simulink model "slexVariantStopCondProp"  (Simulink 10.0)
settings: Solver=FixedStepAuto  StartTime=0.0  StopTime=10.0  RelTol=1e-3  EnableMultiTasking=on
model workspace (MAT data in the model file):
  V = 1
  W : num (value not decoded)
PreLoadFcn:
  | addpath(fileparts(which(bdroot)));
PostLoadFcn:
  | A = Simulink.Parameter(int32(1));
  | A.StorageClass = 'Define (Custom)';
  | A.CoderInfo.CustomAttributes.HeaderFile='variant_defines.h';
  | 
  | W=copy(A);
settings Model: Creator=The MathWorks, Inc.  LastModifiedBy=bhisma
settings DataIOCC: ReturnWorkspaceOutputs=on  OutputSaveName=out1,out2,out3
settings OptimizationCC: LifeSpan=auto
settings DebuggingCC: UnderspecifiedInitializationDetection=Simplified  MergeDetectMultiDrivingBlocksExec=error  PregeneratedLibrarySubsystemCodeDiagnostic=none  SFUnexpectedBacktrackingDiag=error  SFNoUnconditionalDefaultTransitionDiag=error  SFExecutionAtInitializationDiag=warning
settings HardwareCC: ProdBitPerPointer=64  ProdBitPerSizeT=64  ProdBitPerPtrDiffT=64  ProdLargestAtomicFloat=Float  ProdIntDivRoundTo=Zero  ProdEndianess=LittleEndian  ProdWordSize=64  ProdHWDeviceType=Intel->x86-64 (Windows64)
settings ModelReferenceCC: PropagateSignalLabelsOutOfModel=on
settings RTWCC: SystemTargetFile=ert.tlc  TemplateMakefile=ert_default_tmf
settings GRTTargetCC: CombineOutputUpdateFcns=on  GRTInterface=off
settings ConfigComp: CovMetricSettings=dsw  CovShowResultsExplorer=off  CovExternalEMLEnable=off

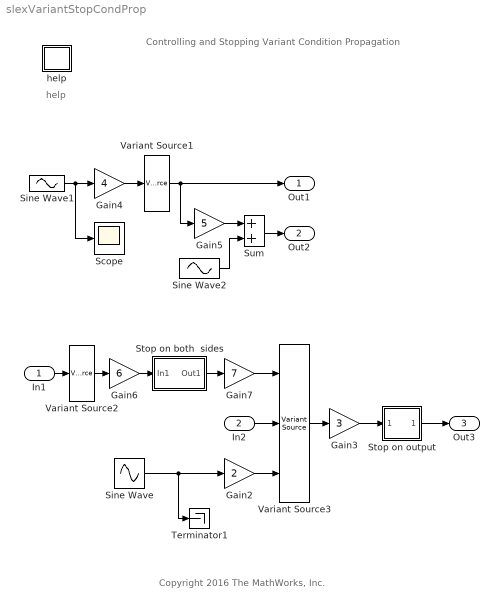
== system slexVariantStopCondProp ==
  note: Controlling and Stopping
      | Variant Condition Propagation
  note: Copyright 2016 The MathWorks, Inc.
  note: help
  In1 : Inport  PortDimensions=1
  In2 : Inport  Port=2  PortDimensions=1
  Gain2 : Gain  Gain=2
  Gain3 : Gain  Gain=3
  Gain4 : Gain  Gain=4
  Gain5 : Gain  Gain=5
  Gain6 : Gain  Gain=6
  Gain7 : Gain  Gain=7
  Scope : Scope
  Sine Wave : Sin  SineType=Sample based  SampleTime=.1
  Sine Wave1 : Sin  SineType=Sample based  SampleTime=.1
  Sine Wave2 : Sin  SineType=Sample based  SampleTime=.1
  Stop on both  sides : Subsystem
  Stop on output : Subsystem
  Sum : Sum
  Terminator1 : Terminator
  Variant Source1 : VariantSource  VariantControls=DataTag1
      settings: GeneratePreprocessorConditionals=on  AllowZeroVariantControls=on
  Variant Source2 : VariantSource  VariantControls=DataTag2
      settings: GeneratePreprocessorConditionals=on  AllowZeroVariantControls=on
  Variant Source3 : VariantSource  VariantControls=DataTag3
      settings: GeneratePreprocessorConditionals=on  AllowZeroVariantControls=on
  help : Subsystem
      mask Display: disp('?')
  Out1 : Outport  VectorParamsAs1DForOutWhenUnconnected=off
  Out2 : Outport  Port=2  VectorParamsAs1DForOutWhenUnconnected=off
  Out3 : Outport  Port=3  VectorParamsAs1DForOutWhenUnconnected=off
  wires:
  Variant Source2/1 -> Gain6/1
  Gain6/1 -> Stop on both  sides/1(In1)
  Stop on both  sides/1(Out1) -> Gain7/1
  Gain7/1 -> Variant Source3/1
  In2/1 -> Variant Source3/2
  Sine Wave/1 -> Terminator1/1, Gain2/1
  Gain2/1 -> Variant Source3/3
  In1/1 -> Variant Source2/1
  Variant Source3/1 -> Gain3/1
  Gain3/1 -> Stop on output/1(In1)
  Stop on output/1(Out1) -> Out3/1
  Sine Wave1/1 -> Gain4/1, Scope/1
  Gain4/1 -> Variant Source1/1
  Sum/1 -> Out2/1
  Sine Wave2/1 -> Sum/2
  Gain5/1 -> Sum/1
  Variant Source1/1 -> Gain5/1, Out1/1

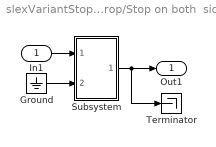
== system slexVariantStopCondProp/Stop on both  sides ==
  In1 : Inport
  Ground : Ground
  Subsystem : Subsystem
  Terminator : Terminator
  Out1 : Outport  VectorParamsAs1DForOutWhenUnconnected=off
  wires:
  In1/1 -> Subsystem/1(In1)
  Ground/1 -> Subsystem/2(In2)
  Subsystem/1(Out1) -> Terminator/1, Out1/1

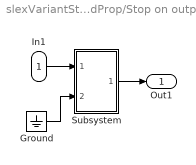
== system slexVariantStopCondProp/Stop on output ==
  In1 : Inport
  Ground : Ground
  Subsystem : Subsystem
  Out1 : Outport  VectorParamsAs1DForOutWhenUnconnected=off
  wires:
  In1/1 -> Subsystem/1(In1)
  Ground/1 -> Subsystem/2(In2)
  Subsystem/1(Out1) -> Out1/1

== system slexVariantStopCondProp/help ==
  note: This illustrates how to control variant condition propagation capabilities of Simulink. Simulink will automatically
      | compute the variant regions based on block connectivity. This is known as variant condition propagation. During
      | variant condition propagation, Simulink automatically assigns conditions to blocks. You can view the conditions
      | assigned to blocks by updating diagram and then looking at the "Display -> Blocks -> Variant Condition Legend".
      |
      | The Variant Source1 has condition, A == 1, which is propagated backwards and forward to the connected blocks. After updating diagram and examining the "Display -> Blocks -> Variant Condition Legend" we see that the Sine Wave1 block is unconditional. This is because the Scope is unconditional and therefore its input, which is the output of the Sine Wave1, must be unconditional. If we were to remove (or comment-out) the Scope, and update diagram we'd see the Sine Wave1 become conditional. Replacing the Scope it with any other block including a Terminator would result in Sine Wave1 being unconditional.
      |
      | We also see that the Sum block is unconditional. This is because the 2nd input to the Sum block is an unconditional signal and therefore the output of the Sum must be unconditional. If we were to place the Gain5, Sum, and Sine Wave2 blocks in a Subsystem (select and ^G) then the Subsystem will be conditional which means the blocks within the Subsystem are also conditional. The subsystem is conditional because it is a system (a well-defined algorithm) with only one input and that input is conditional. If you would like the Subsystem to be treated as an ungrouped collection of blocks and not a system, then you can unselect the "Treat as grouped when propagating variant conditions" parameter in the Subsystem block parameters dialog. This the same as expanding the subsystem in place.
      |
      | We can leverage the properties of variant condition propagation to create stop the propagation. For example, we are using the Terminator1 block to the right to force the Since Wave to always run. Forcing the Sine Wave to be unconditional in this model only means there's unnecessary computation happing. However, you could imagine replacing the Sine Wave with a Subsystem which has dynamics that must always run and the Terminator block can be used to ensure it is not assigned a condition.
      |
      | We can also create a stop propagation block that will stop the variant condition propagation on the output side (stop forward propagation) as shown by the 'Stop on output' block. Note the 'Stop on output' block has the "Treat as grouped when propagating variant conditions" Subsystem parameter turned off.
      |
      | The 'Stop on both sides' stops both forward and backwards propagation by leveraging the properties of variant condition propagation. Again note that the block has the "Treat as grouped when propagating variant conditions" Subsystem parameter turned off.

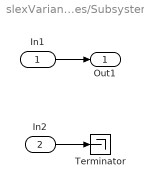
== system slexVariantStopCondProp/Stop on both  sides/Subsystem ==
  In1 : Inport
  In2 : Inport  Port=2
  Terminator : Terminator
  Out1 : Outport  VectorParamsAs1DForOutWhenUnconnected=off
  wires:
  In1/1 -> Out1/1
  In2/1 -> Terminator/1

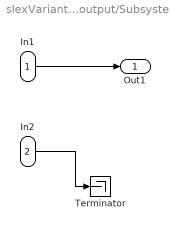
== system slexVariantStopCondProp/Stop on output/Subsystem ==
  In1 : Inport
  In2 : Inport  Port=2
  Terminator : Terminator
  Out1 : Outport  VectorParamsAs1DForOutWhenUnconnected=off
  wires:
  In1/1 -> Out1/1
  In2/1 -> Terminator/1
